simulink model "Lab1_Sim2"  (R2018a)
settings: Solver=FixedStepAuto  StartTime=0.0  StopTime=10  FixedStep=0.002  RelTol=1e-3  EnableMultiTasking=on
settings Model: ExtModeTrigDuration=10000  Creator=nmetzger  LastModifiedBy=nmetzger
settings SolverCC: PositivePriorityOrder=on
settings RTWCC: SystemTargetFile=quarc_win64.tlc  TemplateMakefile=quarc_default_tmf  Description=QUARC Win64 Target
settings STFCustomTargetCC: TargetPreCompLibLocation=C:\PROGRA~3\QUARC\lib\2018a\win64\release  TargetLangStandard=C99 (ISO)  ConcurrentExecutionCompliant=on  SystemTargetFile=quarc_win64.tlc
settings GRTTargetCC: TargetPreCompLibLocation=C:\PROGRA~3\QUARC\lib\2018a\win64\release  ParMdlRefBuildCompliant=off  CompOptLevelCompliant=off  CombineOutputUpdateFcns=off  MatFileLogging=off  CPPClassGenCompliant=off  GRTInterface=on  UseToolchainInfoCompliant=off  ExtMode=on  ExtModeMexFile=quarc_comm

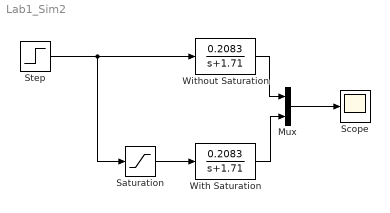
== system Lab1_Sim2 ==
  Mux : Mux  Inputs=2
  Saturation : Saturate  UpperLimit=+5  LowerLimit=-5
  Scope : Scope
  Step : Step  After=10  SampleTime=0
  With Saturation : TransferFcn  Numerator=[0.2083]  Denominator=[1 1.71]
  Without Saturation : TransferFcn  Numerator=[0.2083]  Denominator=[1 1.71]
  wires:
  Step/1 -> Saturation/1, Without Saturation/1
  Without Saturation/1 -> Mux/1
  Saturation/1 -> With Saturation/1
  With Saturation/1 -> Mux/2
  Mux/1 -> Scope/1
